simulink model "mpc_tgt_calc"  (R2025a)
settings: Solver=FixedStepDiscrete  StartTime=0.0  StopTime=2600  FixedStep=0.1  RelTol=1e-3
undefined symbols (not defined in the file): accl, alpha, alpha2, ang, beta, cnt_delay_accl_ratio, cnt_delay_decel_ratio, delay_accl, delay_v, dist, dt, ff_duty_front, ff_duty_l, ff_duty_r, ff_duty_roll, ff_duty_rpm_l, ff_duty_rpm_r, ff_friction_torque_l, ff_friction_torque_r, ff_front_torque, ff_roll_torque, ideal_point, img_ang, img_dist, kanayama_point, pivot_state, pos_x, pos_y, sla_param, slip, slip_point, state, trj_diff, v, vx, vy, w
libraries: simulink_extras x1
(part 3 of 3)

== system mpc_tgt_calc/slalom/Subsystem2/Subsystem/If Action Subsystem2 ==
  Action Port : ActionPort  ActionPortLabel=if(u1 ~= 0)
  Constant1 : Constant  Value=0  OutDataTypeStr=single
  Constant2 : Constant  Value=0  OutDataTypeStr=single
  Mux : Mux  Inputs=2
  Out1 : Outport
  wires:
  Constant2/1 -> Mux/2
  Mux/1 -> Out1/1
  Constant1/1 -> Mux/1

== system mpc_tgt_calc/slalom/Subsystem2/Subsystem/If Action Subsystem3 ==
  ego : Inport
  Action Port : ActionPort  ActionPortLabel=else
  calc_neiper1 : Subsystem
  neipier : Outport
  wires:
  ego/1 -> calc_neiper1/1(ego)
  calc_neiper1/1(neipier) -> neipier/1

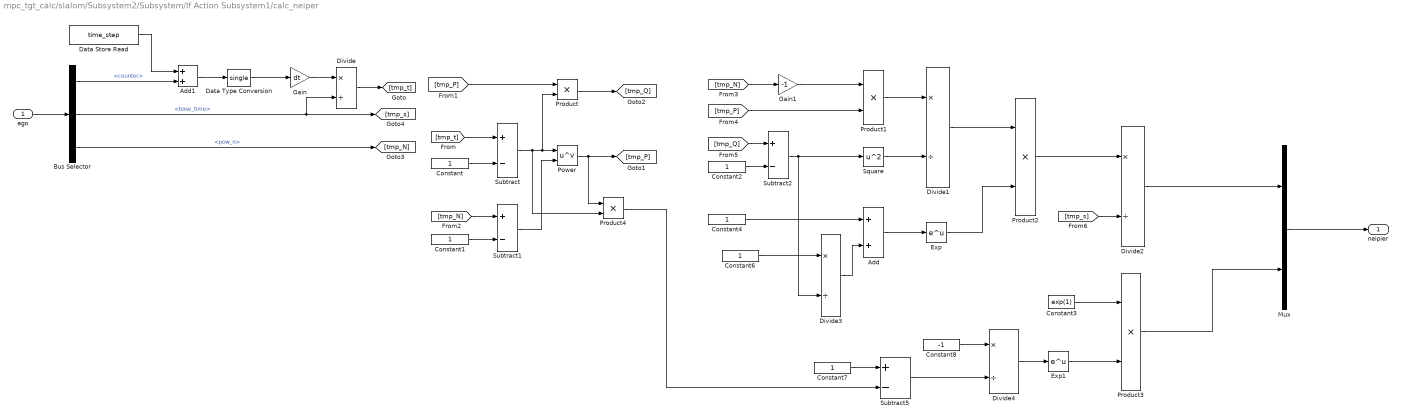
== system mpc_tgt_calc/slalom/Subsystem2/Subsystem/If Action Subsystem1/calc_neiper ==
  ego : Inport
  Add : Sum
  Add1 : Sum
  Bus Selector : BusSelector  OutputSignals=counter,base_time,pow_n
  Constant{,1..2,4,6..7} (6 alike) : Constant  OutDataTypeStr=single
  Constant3 : Constant  Value=exp(1)  OutDataTypeStr=single
  Constant8 : Constant  Value=-1  OutDataTypeStr=single
  Data Store Read : DataStoreRead  DataStoreName=time_step  IndexOptions=Index vector (dialog)  Indices=1  OutputSizes=1
  Data Type Conversion : DataTypeConversion  OutDataTypeStr=single  SaturateOnIntegerOverflow=off  RndMeth=Floor
  Divide{,1..4} (5 alike) : Product  Inputs=*/
  Exp : Math
  Exp1 : Math
  Gain : Gain  Gain=dt
  Gain1 : Gain  Gain=-1
  Mux : Mux  Inputs=2
  Power : Math  Operator=pow
  Product{,1..4} (5 alike) : Product
  Square : Math  Operator=square
  Subtract{,1..2,5} (4 alike) : Sum  Inputs=+-
  neipier : Outport
  wires:
  ego/1 -> Bus Selector/1
  Gain/1 -> Divide/1
  Bus Selector/2 -> Divide/2, [tmp_s]  "<base_time>"
  Divide/1 -> [tmp_t]
  [tmp_t] -> Subtract/1
  Constant/1 -> Subtract/2
  Subtract/1 -> Product4/2, Power/1, Product/2
  Subtract1/1 -> Power/2
  Constant1/1 -> Subtract1/2
  Power/1 -> Product4/1, [tmp_P]
  [tmp_P] -> Product/1
  Product/1 -> [tmp_Q]
  Bus Selector/3 -> [tmp_N]  "<pow_n>"
  [tmp_N] -> Subtract1/1
  [tmp_N] -> Gain1/1
  Gain1/1 -> Product1/1
  [tmp_P] -> Product1/2
  Product1/1 -> Divide1/1
  [tmp_Q] -> Subtract2/1
  Constant2/1 -> Subtract2/2
  Square/1 -> Divide1/2
  Divide1/1 -> Product2/1
  Product2/1 -> Divide2/1
  [tmp_s] -> Divide2/2
  Constant4/1 -> Add/1
  Divide3/1 -> Add/2
  Subtract2/1 -> Divide3/2, Square/1
  Constant6/1 -> Divide3/1
  Add/1 -> Exp/1
  Exp/1 -> Product2/2
  Divide2/1 -> Mux/1
  Bus Selector/1 -> Add1/2  "<counter>"
  Data Type Conversion/1 -> Gain/1
  Data Store Read/1 -> Add1/1
  Add1/1 -> Data Type Conversion/1
  Mux/1 -> neipier/1
  Product4/1 -> Subtract5/2
  Constant7/1 -> Subtract5/1
  Subtract5/1 -> Divide4/2
  Constant8/1 -> Divide4/1
  Divide4/1 -> Exp1/1
  Exp1/1 -> Product3/2
  Constant3/1 -> Product3/1
  Product3/1 -> Mux/2

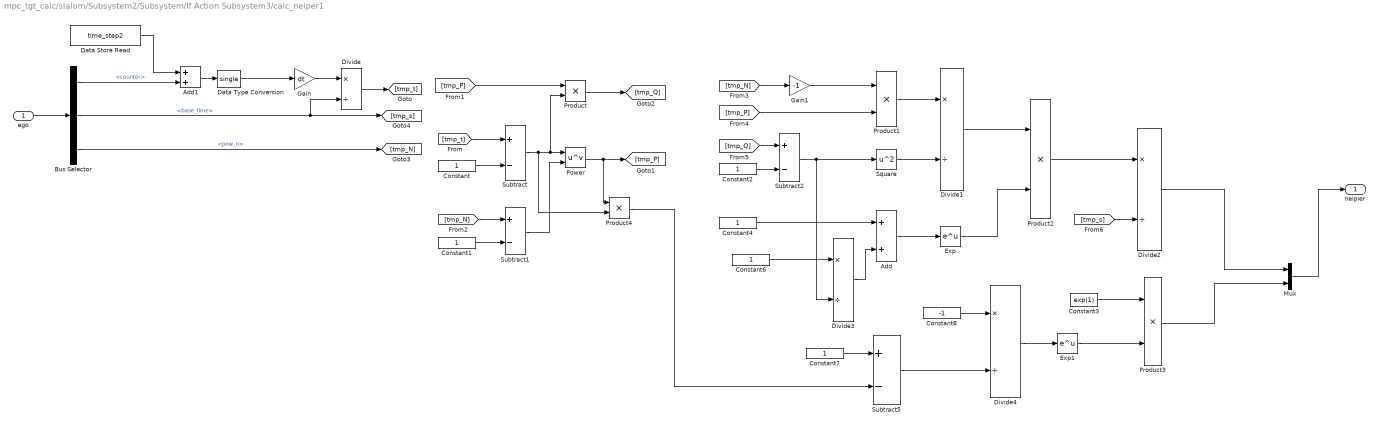
== system mpc_tgt_calc/slalom/Subsystem2/Subsystem/If Action Subsystem3/calc_neiper1 ==
  ego : Inport
  Add : Sum
  Add1 : Sum
  Bus Selector : BusSelector  OutputSignals=counter,base_time,pow_n
  Constant{,1..2,4,6..7} (6 alike) : Constant  OutDataTypeStr=single
  Constant3 : Constant  Value=exp(1)  OutDataTypeStr=single
  Constant8 : Constant  Value=-1  OutDataTypeStr=single
  Data Store Read : DataStoreRead  DataStoreName=time_step2  IndexOptions=Index vector (dialog)  Indices=1  OutputSizes=1
  Data Type Conversion : DataTypeConversion  OutDataTypeStr=single  SaturateOnIntegerOverflow=off  RndMeth=Floor
  Divide{,1..4} (5 alike) : Product  Inputs=*/
  Exp : Math
  Exp1 : Math
  Gain : Gain  Gain=dt
  Gain1 : Gain  Gain=-1
  Mux : Mux  Inputs=2
  Power : Math  Operator=pow
  Product{,1..4} (5 alike) : Product
  Square : Math  Operator=square
  Subtract{,1..2,5} (4 alike) : Sum  Inputs=+-
  neipier : Outport
  wires:
  ego/1 -> Bus Selector/1
  Gain/1 -> Divide/1
  Bus Selector/2 -> Divide/2, [tmp_s]  "<base_time>"
  Divide/1 -> [tmp_t]
  [tmp_t] -> Subtract/1
  Constant/1 -> Subtract/2
  Subtract/1 -> Product4/2, Power/1, Product/2
  Subtract1/1 -> Power/2
  Constant1/1 -> Subtract1/2
  Power/1 -> Product4/1, [tmp_P]
  [tmp_P] -> Product/1
  Product/1 -> [tmp_Q]
  Bus Selector/3 -> [tmp_N]  "<pow_n>"
  [tmp_N] -> Subtract1/1
  [tmp_N] -> Gain1/1
  Gain1/1 -> Product1/1
  [tmp_P] -> Product1/2
  Product1/1 -> Divide1/1
  [tmp_Q] -> Subtract2/1
  Constant2/1 -> Subtract2/2
  Square/1 -> Divide1/2
  Divide1/1 -> Product2/1
  Product2/1 -> Divide2/1
  [tmp_s] -> Divide2/2
  Constant4/1 -> Add/1
  Divide3/1 -> Add/2
  Subtract2/1 -> Divide3/2, Square/1
  Constant6/1 -> Divide3/1
  Add/1 -> Exp/1
  Exp/1 -> Product2/2
  Divide2/1 -> Mux/1
  Bus Selector/1 -> Add1/2  "<counter>"
  Data Type Conversion/1 -> Gain/1
  Data Store Read/1 -> Add1/1
  Add1/1 -> Data Type Conversion/1
  Product3/1 -> Mux/2
  Constant7/1 -> Subtract5/1
  Divide4/1 -> Exp1/1
  Product4/1 -> Subtract5/2
  Subtract5/1 -> Divide4/2
  Constant8/1 -> Divide4/1
  Exp1/1 -> Product3/2
  Constant3/1 -> Product3/1
  Mux/1 -> neipier/1

== matlab function mpc_tgt_calc/kanayama_ctrl_method1/MATLAB Function ==
  data: x output; ego input Bus: t_ego; y output; theta output; tgt input Bus: t_tgt
function [x, y,theta]  = detect_trj_point_impl(ego, tgt)
    [x, y, ~, theta, ~] = detect_trj_point(ego, tgt);
end
